simulink model "simulering_ROV_DP_model"  (R2020a)
settings: Solver=VariableStepAuto  StartTime=0.0  StopTime=t_sim  RelTol=1e-3
values from neighbouring files (symbols this model uses):
  B = [b11 b12 b13 b14 b15 b16 ... (first row only)    [constants.m]    (also in constants_dp_model.m; constants_model_coriolis.m; constants_process_model.m)
  B_psinv = B'/(B*B')    [constants_dp_model.m]    (also in constants_model_coriolis.m)
  d_11 = 250    [constants.m]    (also in constants_dp_model.m; constants_model_coriolis.m; constants_process_model.m)
  d_22 = 200    [constants.m]    (also in constants_dp_model.m; constants_model_coriolis.m; constants_process_model.m)
  d_33 = 175    [constants.m]    (also in constants_dp_model.m; constants_model_coriolis.m; constants_process_model.m)
  d_44 = 20    [constants.m]    (also in constants_dp_model.m = 15; constants_model_coriolis.m = 15; constants_process_model.m)
  g_z = 9.81    [run_simulation_FL_controller.m]    (also in run_simulation_PID_controller.m = 0.91; run_simulation_SM_controller.m = 0.91; run_simulation_STA_controller.m = 0.91; run_simulation_dp_model.m)
  gamma1 = 0.5    [run_simulation_dp_model.m]    (also in tuning_dp_model.m = 50)
  gamma2 = 0.5    [run_simulation_dp_model.m]    (also in tuning_dp_model.m = 35)
  k_d_psi = 2*m_44*zeta_d_psi*wn_psi-d_44    [run_simulation_PID_controller.m]    (also in run_simulation_SM_controller.m = 10; run_simulation_dp_model.m; run_simulation_feedback_linearizing.m = (2*1*k_p_psi*1-d33/(m_A33+m_RB33)); tuning_PID_controller.m = 2*m_66*zeta_d_psi*wn_psi-d_66)
  k_d_w = 2*m_33*zeta_d_heave*wn_heave-d_33    [run_simulation_FL_controller.m]    (also in run_simulation_dp_model.m; run_simulation_feedback_linearizing_second_try.m)
  k_i_psi = wn_psi/10*k_p_psi    [run_simulation_PID_controller.m]    (also in run_simulation_dp_model.m = 1/10*k_p_psi; tuning_PID_controller.m; tuning_dp_model.m = 0)
  k_i_w = wn_heave/10*k_p_w    [run_simulation_FL_controller.m]    (also in run_simulation_dp_model.m; run_simulation_feedback_linearizing_second_try.m)
  k_p_psi = wn_psi^2-lambda*k_p_r    [run_simulation_FL_controller.m]    (also in run_simulation_PID_controller.m = wn_psi^2*m_44; run_simulation_dp_model.m = wn_psi^2*m_44; run_simulation_feedback_linearizing.m = tau_r_max/deg2rad(45); run_simulation_feedback_linearizing_second_try.m = wn_psi^2*m_44)
  k_p_u = m_11*pole_u-d_11    [run_simulation_FL_controller.m]    (also in run_simulation_PID_controller.m = 10; run_simulation_dp_model.m = pole_u-d_11/m_11; run_simulation_feedback_linearizing.m = tau_u_max/100; run_simulation_feedback_linearizing_second_try.m = 1)
  k_p_v = m_22*pole_v-d_22    [run_simulation_FL_controller.m]    (also in run_simulation_PID_controller.m = 10; run_simulation_dp_model.m = pole_v-d_22/m_22; run_simulation_feedback_linearizing.m = tau_v_max/100; run_simulation_feedback_linearizing_second_try.m = 1)
  k_p_w = wn_heave^2*m_33    [run_simulation_FL_controller.m]    (also in run_simulation_dp_model.m; run_simulation_feedback_linearizing_second_try.m)
  m_11 = m_RB11+m_A11    (= 144)    [constants.m]    (also in constants_dp_model.m; constants_model_coriolis.m; constants_process_model.m)
  m_22 = m_RB22+m_A22    (= 162)    [constants.m]    (also in constants_dp_model.m; constants_model_coriolis.m; constants_process_model.m)
  m_A11 = 54    [constants.m]    (also in constants_dp_model.m; constants_model_coriolis.m; constants_process_model.m)
  m_A22 = 72    [constants.m]    (also in constants_dp_model.m; constants_model_coriolis.m; constants_process_model.m)
  m_A33 = 360    [constants.m]    (also in constants_dp_model.m; constants_model_coriolis.m; constants_process_model.m)
  m_A44 = 11    [constants.m]    (also in constants_dp_model.m = 5.2; constants_model_coriolis.m = 5.2; constants_process_model.m)
  m_RB11 = 90    [constants.m]    (also in constants_dp_model.m; constants_model_coriolis.m; constants_process_model.m)
  m_RB22 = 90    [constants.m]    (also in constants_dp_model.m; constants_model_coriolis.m; constants_process_model.m)
  m_RB33 = 90    [constants.m]    (also in constants_dp_model.m; constants_model_coriolis.m; constants_process_model.m)
  m_RB44 = 10    [constants.m]    (also in constants_dp_model.m = 13; constants_model_coriolis.m = 13; constants_process_model.m)
  omega_ref = 1.5    [run_simulation.m]    (also in run_simulation_FL_controller.m = 0.4; run_simulation_PID_controller.m = 0.4; run_simulation_SM_controller.m; run_simulation_STA_controller.m)
  psi0 = deg2rad(psi0)    [constants.m]    (also in constants_dp_model.m; constants_model_coriolis.m; constants_process_model.m)
  psi_r1 = deg2rad(psi_r1)    [run_simulation.m]    (also in run_simulation_FL_controller.m = 45; run_simulation_PID_controller.m = 45; run_simulation_SM_controller.m; run_simulation_STA_controller.m)
  psi_r2 = deg2rad(psi_r2)    [run_simulation.m]    (also in run_simulation_FL_controller.m = 90; run_simulation_PID_controller.m = 90; run_simulation_SM_controller.m; run_simulation_STA_controller.m)
  r0 = 0    [constants.m]    (also in constants_dp_model.m; constants_model_coriolis.m; constants_process_model.m)
  T_ref = 0.2    [run_simulation.m]    (also in run_simulation_FL_controller.m; run_simulation_PID_controller.m; run_simulation_SM_controller.m; run_simulation_STA_controller.m)
  tau_r_max = sqrt(torque_co'*torque_co)    [constants.m]    (also in constants_dp_model.m; constants_model_coriolis.m; constants_process_model.m; run_simulation_feedback_linearizing.m = sqrt(torque_co'*torque_co)/(m_A33+m_RB33))
  tau_u_max = (F_max*cos(alpha1)+F_max*cos(alpha2)+F_max*cos(alpha3)+F_max*cos(alpha4))    [constants.m]    (also in constants_dp_model.m; constants_model_coriolis.m; constants_process_model.m; run_simulation_feedback_linearizing.m = (F_max*cos(alpha1)+F_max*cos(alpha2)+F_max*cos(alpha3)+F_max)
  tau_v_max = (F_max*sin(alpha1)-F_max*sin(alpha2)+F_max*sin(alpha3)-F_max*sin(alpha4))    [constants.m]    (also in constants_dp_model.m; constants_model_coriolis.m; constants_process_model.m; run_simulation_feedback_linearizing.m = (F_max*sin(alpha1)-F_max*sin(alpha2)+F_max*sin(alpha3)-F_max)
  tau_w_max = 2*F_max    (= 240)    [constants.m]    (also in constants_dp_model.m; constants_model_coriolis.m; constants_process_model.m)
  u0 = 0    [constants.m]    (also in constants_dp_model.m; constants_model_coriolis.m; constants_process_model.m)
  u_r = 0.14    [run_simulation.m]    (also in run_simulation_FL_controller.m = 0.2; run_simulation_PID_controller.m = 0.2; run_simulation_SM_controller.m; run_simulation_STA_controller.m)
  v0 = 0    [constants.m]    (also in constants_dp_model.m; constants_model_coriolis.m; constants_process_model.m)
  v_r = 0.14    [run_simulation.m]    (also in run_simulation_FL_controller.m = 0; run_simulation_PID_controller.m = 0; run_simulation_SM_controller.m; run_simulation_STA_controller.m)
  V_x = 1    [constants.m]    (also in constants_process_model.m; run_simulation_FL_controller.m = 0.25; run_simulation_PID_controller.m = 0.25; run_simulation_dp_model.m = 0.25)
  V_y = 0    [constants.m]    (also in constants_process_model.m; run_simulation_FL_controller.m = -0.6; run_simulation_PID_controller.m = -0.6; run_simulation_dp_model.m = -0.6)
  w0 = 0    [constants.m]    (also in constants_dp_model.m; constants_model_coriolis.m; constants_process_model.m)
  x0 = -2*50    (= -100)    [constants.m]    (also in constants_dp_model.m = 0; constants_model_coriolis.m = 0; constants_process_model.m = 0)
  y0 = 0    [constants.m]    (also in constants_dp_model.m; constants_model_coriolis.m; constants_process_model.m)
  z0 = 0    [constants.m]    (also in constants_dp_model.m; constants_model_coriolis.m; constants_process_model.m)
  z_r = 10    [run_simulation.m]    (also in run_simulation_FL_controller.m = 1; run_simulation_PID_controller.m = 1; run_simulation_SM_controller.m; run_simulation_STA_controller.m)
  zeta_ref = 1    [run_simulation.m]    (also in run_simulation_FL_controller.m; run_simulation_PID_controller.m; run_simulation_SM_controller.m; run_simulation_STA_controller.m)
settings Model: Creator=kenng  LastModifiedBy=kenng

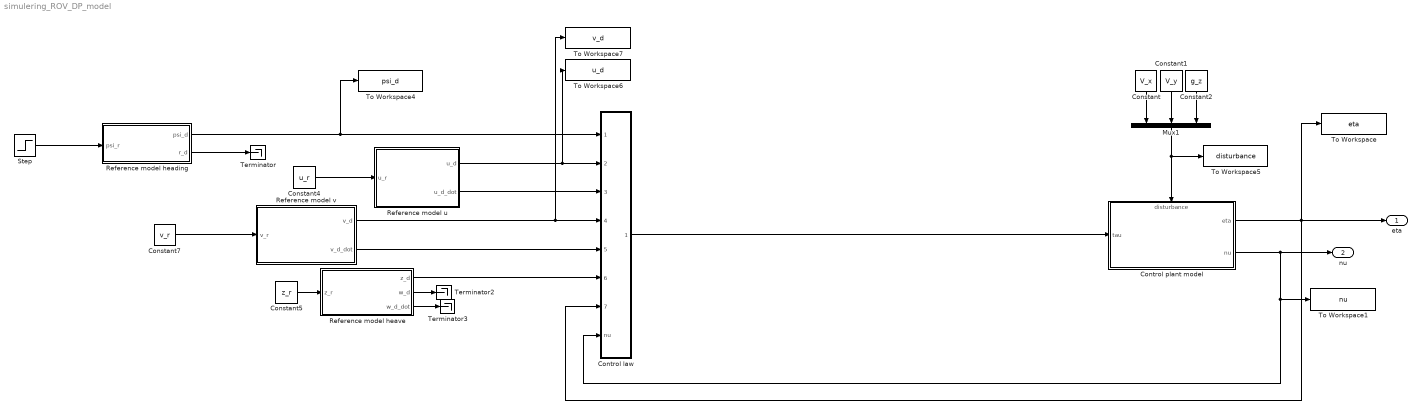
== system simulering_ROV_DP_model ==
  Constant : Constant  Value=V_x
  Constant1 : Constant  Value=V_y
  Constant2 : Constant  Value=g_z
  Constant4 : Constant  Value=u_r
  Constant5 : Constant  Value=z_r
  Constant7 : Constant  Value=v_r
  Control law : Subsystem
  Control plant model : Subsystem
      settings: PortSchema="{\"entries\":[{\"content\":{\"sides\":[{\"content\":{\"connectorIds\":[\"In1\"]},\"type\":\"ConnectorPlacement.EquallySpacedRectSide\",\"uuid\":\"e717a587-3200-458e-ba24-dd41565550b9\"},{\"content\":{\"connectorIds\":[\"Out1\",\"Out2\"],\"side\":\"RIGHT\"},\"type\":\"ConnectorPlacement.EquallySpacedRectSide\",\"uuid\":\"302c9cc9-c34e-45c2-bf93-40982187bd66\"},{\"content\":{\"connectorIds\":[\"In2\"],\"side\":\"TOP\"},\"type\":\"ConnectorPlacement.EquallySpacedRectSide\",\"uuid\":\"4b1c13ad-6fa1-447d-8a08-ad292496a8ea\"}]},\"type\":\"ConnectorPlacement.EquallySpacedConnector\",\"uuid\":\"78ff5622-69b9-4402-ac71-5e2cc2861626\"}],\"packageUris\":[\"http://schema.mathworks.com/mf0/Connector/19700101\"],\"version\":\"1.0\"}"
  Mux1 : Mux  Inputs=3
  Reference model heading : Subsystem
  Reference model heave : Subsystem
  Reference model u : Subsystem
  Reference model v : Subsystem
  Step : Step  Time=1000  Before=deg2rad(psi_r1)  After=deg2rad(psi_r2)  SampleTime=0
  Terminator : Terminator
  Terminator2 : Terminator
  Terminator3 : Terminator
  To Workspace : ToWorkspace  VariableName=eta  SaveFormat=Structure With Time  SampleTime=-1
  To Workspace1 : ToWorkspace  VariableName=nu  SaveFormat=Structure With Time  SampleTime=-1
  To Workspace4 : ToWorkspace  VariableName=psi_d  SaveFormat=Structure With Time  SampleTime=-1
  To Workspace5 : ToWorkspace  VariableName=disturbance  SaveFormat=Structure With Time  SampleTime=-1
  To Workspace6 : ToWorkspace  VariableName=u_d  SaveFormat=Structure With Time  SampleTime=-1
  To Workspace7 : ToWorkspace  VariableName=v_d  SaveFormat=Structure With Time  SampleTime=-1
  eta : Outport
  nu : Outport  Port=2
  wires:
  Control plant model/1(eta) -> Control law/7(eta), eta/1, To Workspace/1
  Control plant model/2(nu) -> nu/1, To Workspace1/1, Control law/8(nu)
  Mux1/1 -> Control plant model/2(disturbance), To Workspace5/1
  Reference model heading/1(psi_d) -> Control law/1(psi_d), To Workspace4/1
  Constant/1 -> Mux1/1
  Constant1/1 -> Mux1/2
  Constant2/1 -> Mux1/3
  Reference model heave/1(z_d) -> Control law/6(z_d)
  Control law/1(tau) -> Control plant model/1(tau)
  Step/1 -> Reference model heading/1(psi_r)
  Reference model heading/2(r_d) -> Terminator/1
  Constant4/1 -> Reference model u/1(u_r)
  Reference model heave/3(w_d_dot) -> Terminator3/1
  Reference model heave/2(w_d) -> Terminator2/1
  Constant5/1 -> Reference model heave/1(z_r)
  Constant7/1 -> Reference model v/1(v_r)
  Reference model u/1(u_d) -> To Workspace6/1, Control law/2(u_d)
  Reference model u/2(u_d_dot) -> Control law/3(u_d_dot)
  Reference model v/1(v_d) -> To Workspace7/1, Control law/4(v_d)
  Reference model v/2(v_d_dot) -> Control law/5(v_d_dot)

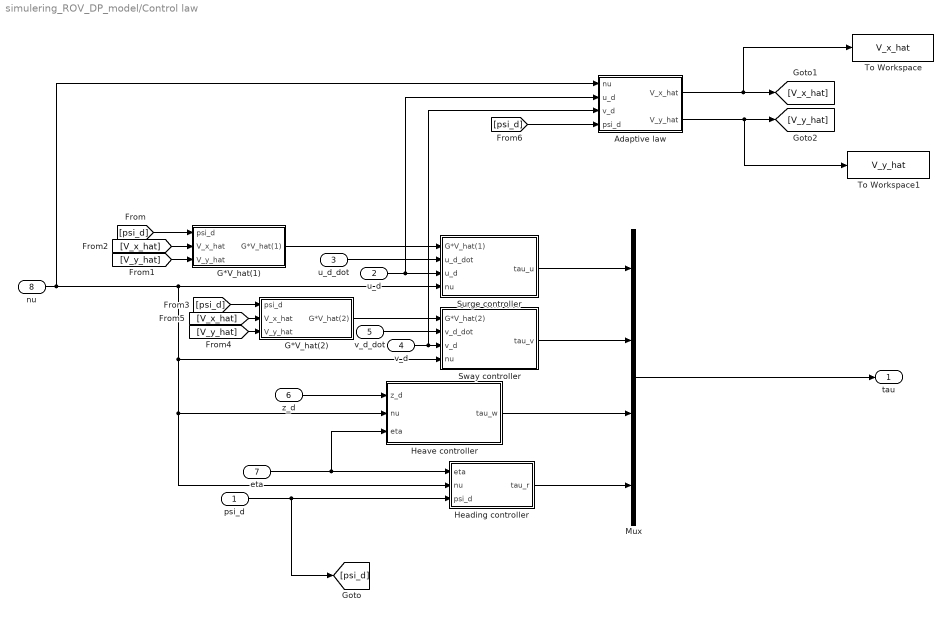
== system simulering_ROV_DP_model/Control law ==
  psi_d : Inport
  u_d : Inport  Port=2
  u_d_dot : Inport  Port=3
  v_d : Inport  Port=4
  v_d_dot : Inport  Port=5
  z_d : Inport  Port=6
  eta : Inport  Port=7
  nu : Inport  Port=8
  Adaptive law : Subsystem
  G*V_hat(1) : Subsystem
  G*V_hat(2) : Subsystem
  Heading controller : Subsystem
  Heave controller : Subsystem
  Mux : Mux
  Surge controller : Subsystem
  Sway controller : Subsystem
  To Workspace : ToWorkspace  VariableName=V_x_hat  SaveFormat=Structure With Time  SampleTime=-1
  To Workspace1 : ToWorkspace  VariableName=V_y_hat  SaveFormat=Structure With Time  SampleTime=-1
  tau : Outport
  wires:
  Surge controller/1(tau_u) -> Mux/1
  Sway controller/1(tau_v) -> Mux/2
  Heave controller/1(tau_w) -> Mux/3
  Mux/1 -> tau/1
  Heading controller/1(tau_r) -> Mux/4
  nu/1 -> Adaptive law/1(nu), Sway controller/4(nu), Heading controller/2(nu), Heave controller/2(nu), Surge controller/4(nu)
  eta/1 -> Heading controller/1(eta), Heave controller/3(eta)
  psi_d/1 -> [psi_d], Heading controller/3(psi_d)
  [V_y_hat] -> G*V_hat(1)/3(V_y_hat)
  [V_x_hat] -> G*V_hat(1)/2(V_x_hat)
  [psi_d] -> G*V_hat(1)/1(psi_d)
  G*V_hat(1)/1(G*V_hat(1)) -> Surge controller/1(G*V_hat(1))
  [psi_d] -> G*V_hat(2)/1(psi_d)
  [V_y_hat] -> G*V_hat(2)/3(V_y_hat)
  [V_x_hat] -> G*V_hat(2)/2(V_x_hat)
  G*V_hat(2)/1(G*V_hat(2)) -> Sway controller/1(G*V_hat(2))
  u_d/1 -> Adaptive law/2(u_d), Surge controller/3(u_d)
  u_d_dot/1 -> Surge controller/2(u_d_dot)
  v_d_dot/1 -> Sway controller/2(v_d_dot)
  v_d/1 -> Adaptive law/3(v_d), Sway controller/3(v_d)
  Adaptive law/1(V_x_hat) -> To Workspace/1, [V_x_hat]
  Adaptive law/2(V_y_hat) -> To Workspace1/1, [V_y_hat]
  [psi_d] -> Adaptive law/4(psi_d)
  z_d/1 -> Heave controller/1(z_d)

== system simulering_ROV_DP_model/Control plant model ==
  note: tau: 4x1 vector = [surge sway heave yaw]^T
  note: Disturbance: 3x1 vector = [Vx Vy gz]^t
  tau : Inport
  disturbance : Inport  Port=2
  Demux : Demux
  Kinematics : Subsystem
  Kinetics : Subsystem
  Terminator : Terminator
  Terminator1 : Terminator
  Terminator2 : Terminator
  Thruster saturation : Subsystem
  To Workspace2 : ToWorkspace  VariableName=tau_unsat  SaveFormat=Structure With Time  SampleTime=-1
  To Workspace3 : ToWorkspace  VariableName=tau_sat  SaveFormat=Structure With Time  SampleTime=-1
  eta : Outport
  nu : Outport  Port=2
  wires:
  Kinetics/1(nu) -> nu/1, Kinematics/1(nu)
  Demux/4 -> Kinetics/3(psi)
  Demux/2 -> Terminator1/1
  Kinematics/1(eta) -> eta/1, Demux/1
  Demux/1 -> Terminator/1
  Demux/3 -> Terminator2/1
  disturbance/1 -> Kinetics/1(disturbance)
  tau/1 -> To Workspace2/1, Thruster saturation/1(tau_unsat)
  Thruster saturation/1(tau_sat) -> To Workspace3/1, Kinetics/2(tau)

== system simulering_ROV_DP_model/Reference model heading ==
  note: psi_r
  note: psi_d
  note: r_d
  note: a_d
  psi_r : Inport
  Gain : Gain  Gain=(2*zeta_ref+1)*omega_ref
  Gain1 : Gain  Gain=(2*zeta_ref+1)*omega_ref^2
  Gain2 : Gain  Gain=omega_ref^3
  Integrator : Integrator
  Integrator1 : Integrator
  Integrator2 : Integrator
  Saturation : Saturate  UpperLimit=tau_r_max/(m_RB11*0.2^2)  LowerLimit=-tau_r_max/(m_RB11*0.2^2)
  Sum : Sum  Inputs=|+-
  Sum1 : Sum  Inputs=-+|
  Sum2 : Sum  Inputs=-+|
  psi_d : Outport
  r_d : Outport  Port=2
  wires:
  Sum1/1 -> Integrator1/1
  Sum2/1 -> Gain2/1
  Integrator2/1 -> psi_d/1, Sum2/1
  Sum/1 -> Sum1/2
  Saturation/1 -> Gain/1, Integrator/1
  Integrator/1 -> r_d/1, Gain1/1, Integrator2/1
  Gain2/1 -> Sum/1
  Gain/1 -> Sum/2
  Gain1/1 -> Sum1/1
  Integrator1/1 -> Saturation/1
  psi_r/1 -> Sum2/2

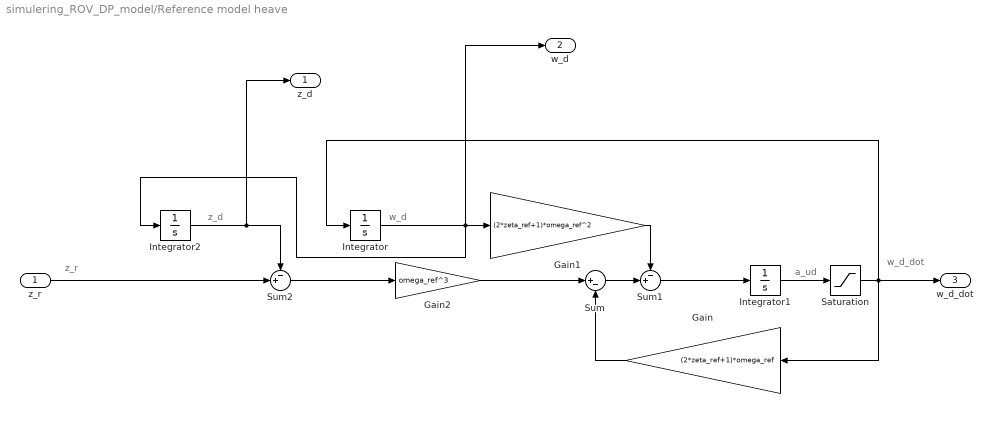
== system simulering_ROV_DP_model/Reference model heave ==
  note: w_d_dot
  note: z_r
  note: z_d
  note: w_d
  note: a_ud
  z_r : Inport
  Gain : Gain  Gain=(2*zeta_ref+1)*omega_ref
  Gain1 : Gain  Gain=(2*zeta_ref+1)*omega_ref^2
  Gain2 : Gain  Gain=omega_ref^3
  Integrator : Integrator
  Integrator1 : Integrator
  Integrator2 : Integrator
  Saturation : Saturate  UpperLimit=tau_w_max/m_RB11  LowerLimit=-tau_w_max/m_RB11
  Sum : Sum  Inputs=|+-
  Sum1 : Sum  Inputs=-+|
  Sum2 : Sum  Inputs=-+|
  z_d : Outport
  w_d : Outport  Port=2
  w_d_dot : Outport  Port=3
  wires:
  Sum1/1 -> Integrator1/1
  Sum2/1 -> Gain2/1
  Integrator2/1 -> z_d/1, Sum2/1
  Sum/1 -> Sum1/2
  Saturation/1 -> Integrator/1, w_d_dot/1, Gain/1
  Gain2/1 -> Sum/1
  Gain/1 -> Sum/2
  Gain1/1 -> Sum1/1
  Integrator1/1 -> Saturation/1
  z_r/1 -> Sum2/2
  Integrator/1 -> w_d/1, Gain1/1, Integrator2/1

== system simulering_ROV_DP_model/Reference model u ==
  note: u_r
  u_r : Inport
  Gain : Gain  Gain=1/T_ref
  Integrator : Integrator
  Saturation : Saturate  UpperLimit=tau_u_max/m_RB11  LowerLimit=-tau_u_max/m_RB11
  Sum : Sum  Inputs=|+-
  u_d : Outport
  u_d_dot : Outport  Port=2
  wires:
  u_r/1 -> Sum/1
  Sum/1 -> Gain/1
  Integrator/1 -> u_d/1, Sum/2
  Gain/1 -> Saturation/1
  Saturation/1 -> u_d_dot/1, Integrator/1

== system simulering_ROV_DP_model/Reference model v ==
  note: v_r
  v_r : Inport
  Gain : Gain  Gain=1/T_ref
  Integrator : Integrator
  Saturation : Saturate
  Saturation1 : Saturate  UpperLimit=tau_v_max/m_RB11  LowerLimit=-tau_v_max/m_RB11
  Sum : Sum  Inputs=|+-
  v_d : Outport
  v_d_dot : Outport  Port=2
  wires:
  v_r/1 -> Sum/1
  Sum/1 -> Gain/1
  Integrator/1 -> Saturation/1
  Gain/1 -> Saturation1/1
  Saturation/1 -> v_d/1, Sum/2
  Saturation1/1 -> v_d_dot/1, Integrator/1

== system simulering_ROV_DP_model/Control law/Adaptive law ==
  nu : Inport
  u_d : Inport  Port=2
  v_d : Inport  Port=3
  psi_d : Inport  Port=4
  Subsystem : Subsystem
  v_x_hat : Subsystem
  v_y_hat : Subsystem
  V_x_hat : Outport
  V_y_hat : Outport  Port=2
  wires:
  nu/1 -> Subsystem/1(nu)
  Subsystem/2(v_tilde) -> v_y_hat/3(v_tilde), v_x_hat/3(v_tilde)
  psi_d/1 -> v_y_hat/1(psi_d), v_x_hat/1(psi_d)
  Subsystem/1(u_tilde) -> v_x_hat/2(u_tilde), v_y_hat/2(u_tilde)
  v_d/1 -> Subsystem/3(v_d)
  v_x_hat/1(V_x_hat) -> V_x_hat/1
  u_d/1 -> Subsystem/2(u_d)
  v_y_hat/1(V_y_hat) -> V_y_hat/1

== system simulering_ROV_DP_model/Control law/G*V_hat(1) ==
  psi_d : Inport
  V_x_hat : Inport  Port=2
  V_y_hat : Inport  Port=3
  Cos : Trigonometry  Operator=cos
  Gain : Gain  Gain=d_11/m_11
  Gain1 : Gain  Gain=d_11/m_11
  Product : Product
  Product1 : Product
  Sin : Trigonometry
  Sum : Sum  Inputs=|++
  G*V_hat(1) : Outport
  wires:
  Gain1/1 -> Product1/1
  Sin/1 -> Gain1/1
  psi_d/1 -> Sin/1, Cos/1
  Product/1 -> Sum/1
  Product1/1 -> Sum/2
  V_x_hat/1 -> Product/1
  Cos/1 -> Gain/1
  V_y_hat/1 -> Product1/2
  Gain/1 -> Product/2
  Sum/1 -> G*V_hat(1)/1

== system simulering_ROV_DP_model/Control law/G*V_hat(2) ==
  psi_d : Inport
  V_x_hat : Inport  Port=2
  V_y_hat : Inport  Port=3
  Cos : Trigonometry  Operator=cos
  Gain : Gain  Gain=d_22/m_22
  Gain1 : Gain  Gain=d_22/m_22
  Product : Product
  Product1 : Product
  Sin : Trigonometry
  Sum : Sum  Inputs=|+-
  G*V_hat(2) : Outport
  wires:
  Sum/1 -> G*V_hat(2)/1
  Gain/1 -> Product/2
  V_x_hat/1 -> Product1/2
  Cos/1 -> Gain/1
  V_y_hat/1 -> Product/1
  Product1/1 -> Sum/2
  Product/1 -> Sum/1
  psi_d/1 -> Cos/1, Sin/1
  Sin/1 -> Gain1/1
  Gain1/1 -> Product1/1

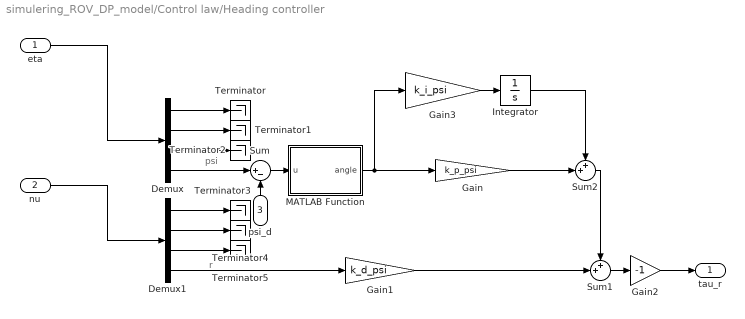
== system simulering_ROV_DP_model/Control law/Heading controller ==
  note: r
  note: psi
  eta : Inport
  nu : Inport  Port=2
  psi_d : Inport  Port=3
  Demux : Demux
  Demux1 : Demux
  Gain : Gain  Gain=k_p_psi
  Gain1 : Gain  Gain=k_d_psi
  Gain2 : Gain  Gain=-1
  Gain3 : Gain  Gain=k_i_psi
  Integrator : Integrator
  MATLAB Function : MATLAB Function  TreatAsAtomicUnit=on
  Sum : Sum  Inputs=|+-
  Sum1 : Sum  Inputs=++|
  Sum2 : Sum  Inputs=++|
  Terminator{,1..5} (6 alike) : Terminator
  tau_r : Outport
  wires:
  Demux1/2 -> Terminator4/1
  Demux/3 -> Terminator2/1
  Demux1/1 -> Terminator3/1
  Gain1/1 -> Sum1/2
  Demux/1 -> Terminator/1
  Sum1/1 -> Gain2/1
  Demux/2 -> Terminator1/1
  Demux1/4 -> Gain1/1
  Demux1/3 -> Terminator5/1
  Demux/4 -> Sum/1
  Sum/1 -> MATLAB Function/1(u)
  eta/1 -> Demux/1
  Gain2/1 -> tau_r/1
  nu/1 -> Demux1/1
  psi_d/1 -> Sum/2
  MATLAB Function/1(angle) -> Gain/1, Gain3/1
  Gain3/1 -> Integrator/1
  Gain/1 -> Sum2/2
  Sum2/1 -> Sum1/1
  Integrator/1 -> Sum2/1

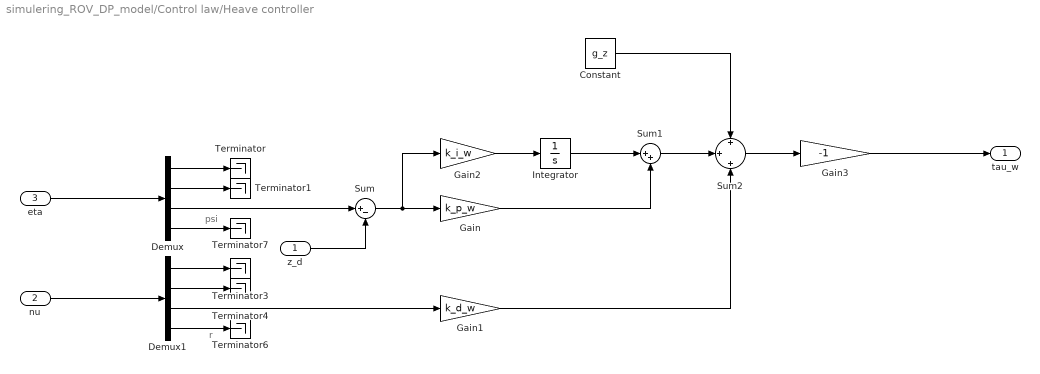
== system simulering_ROV_DP_model/Control law/Heave controller ==
  note: r
  note: psi
  z_d : Inport
  nu : Inport  Port=2
  eta : Inport  Port=3
  Constant : Constant  Value=g_z
  Demux : Demux
  Demux1 : Demux
  Gain : Gain  Gain=k_p_w
  Gain1 : Gain  Gain=k_d_w
  Gain2 : Gain  Gain=k_i_w
  Gain3 : Gain  Gain=-1
  Integrator : Integrator
  Sum : Sum  Inputs=|+-
  Sum1 : Sum  Inputs=|++
  Sum2 : Sum  Inputs=+|+|+
  Terminator{,1,3..4,6..7} (6 alike) : Terminator
  tau_w : Outport
  wires:
  Demux1/2 -> Terminator4/1
  Demux/1 -> Terminator/1
  eta/1 -> Demux/1
  Demux/2 -> Terminator1/1
  Demux1/1 -> Terminator3/1
  Demux/3 -> Sum/1
  nu/1 -> Demux1/1
  Demux1/4 -> Terminator6/1
  Demux/4 -> Terminator7/1
  z_d/1 -> Sum/2
  Sum/1 -> Gain2/1, Gain/1
  Demux1/3 -> Gain1/1
  Gain2/1 -> Integrator/1
  Integrator/1 -> Sum1/1
  Gain/1 -> Sum1/2
  Sum2/1 -> Gain3/1
  Gain3/1 -> tau_w/1
  Gain1/1 -> Sum2/3
  Sum1/1 -> Sum2/2
  Constant/1 -> Sum2/1

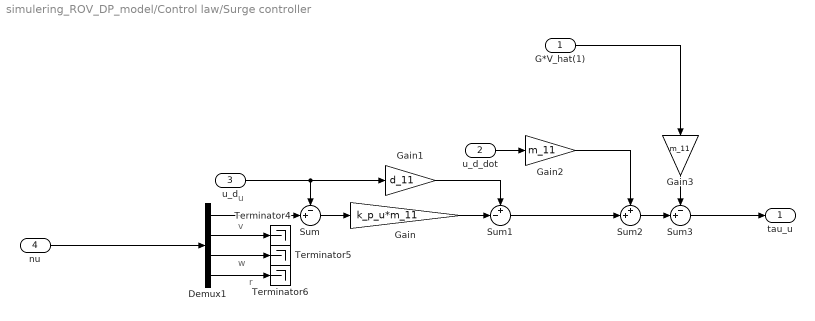
== system simulering_ROV_DP_model/Control law/Surge controller ==
  note: u
  note: r
  note: v
  note: w
  G*V_hat(1) : Inport
  u_d_dot : Inport  Port=2
  u_d : Inport  Port=3
  nu : Inport  Port=4
  Demux1 : Demux
  Gain : Gain  Gain=k_p_u*m_11
  Gain1 : Gain  Gain=d_11
  Gain2 : Gain  Gain=m_11
  Gain3 : Gain  Gain=m_11
  Sum : Sum  Inputs=-+|
  Sum1 : Sum  Inputs=+-|
  Sum2 : Sum  Inputs=++|
  Sum3 : Sum  Inputs=-+|
  Terminator4 : Terminator
  Terminator5 : Terminator
  Terminator6 : Terminator
  tau_u : Outport
  wires:
  Demux1/2 -> Terminator4/1
  Demux1/4 -> Terminator6/1
  Demux1/1 -> Sum/2
  nu/1 -> Demux1/1
  Demux1/3 -> Terminator5/1
  u_d/1 -> Gain1/1, Sum/1
  Sum/1 -> Gain/1
  Gain/1 -> Sum1/2
  Gain1/1 -> Sum1/1
  Sum1/1 -> Sum2/2
  u_d_dot/1 -> Gain2/1
  Gain2/1 -> Sum2/1
  Sum2/1 -> Sum3/2
  Gain3/1 -> Sum3/1
  G*V_hat(1)/1 -> Gain3/1
  Sum3/1 -> tau_u/1

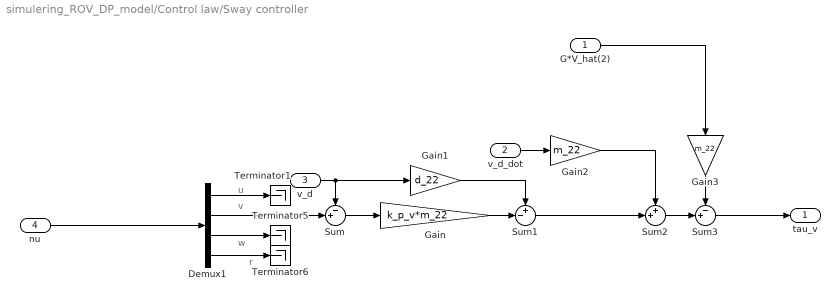
== system simulering_ROV_DP_model/Control law/Sway controller ==
  note: w
  note: v
  note: r
  note: u
  G*V_hat(2) : Inport
  v_d_dot : Inport  Port=2
  v_d : Inport  Port=3
  nu : Inport  Port=4
  Demux1 : Demux
  Gain : Gain  Gain=k_p_v*m_22
  Gain1 : Gain  Gain=d_22
  Gain2 : Gain  Gain=m_22
  Gain3 : Gain  Gain=m_22
  Sum : Sum  Inputs=-+|
  Sum1 : Sum  Inputs=+-|
  Sum2 : Sum  Inputs=++|
  Sum3 : Sum  Inputs=-+|
  Terminator1 : Terminator
  Terminator5 : Terminator
  Terminator6 : Terminator
  tau_v : Outport
  wires:
  Sum3/1 -> tau_v/1
  G*V_hat(2)/1 -> Gain3/1
  Gain3/1 -> Sum3/1
  Sum2/1 -> Sum3/2
  Gain2/1 -> Sum2/1
  v_d_dot/1 -> Gain2/1
  Sum1/1 -> Sum2/2
  Gain1/1 -> Sum1/1
  Gain/1 -> Sum1/2
  Sum/1 -> Gain/1
  v_d/1 -> Sum/1, Gain1/1
  Demux1/3 -> Terminator5/1
  nu/1 -> Demux1/1
  Demux1/4 -> Terminator6/1
  Demux1/2 -> Sum/2
  Demux1/1 -> Terminator1/1

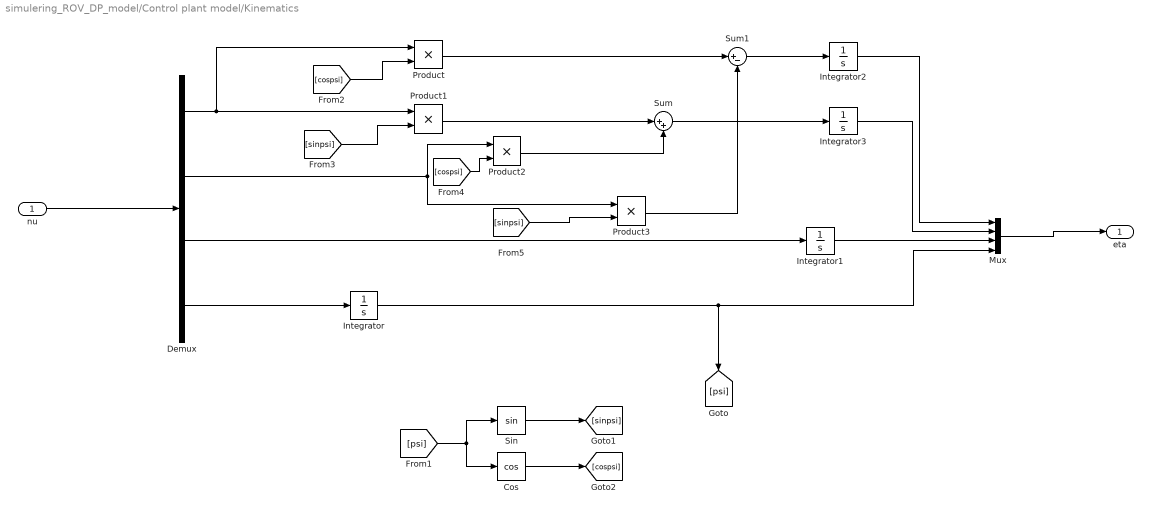
== system simulering_ROV_DP_model/Control plant model/Kinematics ==
  nu : Inport
  Cos : Trigonometry  Operator=cos
  Demux : Demux
  Integrator : Integrator  InitialCondition=psi0
  Integrator1 : Integrator  InitialCondition=z0
  Integrator2 : Integrator  InitialCondition=x0
  Integrator3 : Integrator  InitialCondition=y0
  Mux : Mux
  Product{,1..3} (4 alike) : Product
  Sin : Trigonometry
  Sum : Sum  Inputs=|++
  Sum1 : Sum  Inputs=|+-
  eta : Outport
  wires:
  Sin/1 -> [sinpsi]
  Demux/3 -> Integrator1/1
  Demux/1 -> Product1/1, Product/1
  Demux/2 -> Product3/1, Product2/1
  [sinpsi] -> Product3/2
  [psi] -> Sin/1, Cos/1
  [cospsi] -> Product2/2
  Cos/1 -> [cospsi]
  Product1/1 -> Sum/1
  Integrator/1 -> Mux/4, [psi]
  [sinpsi] -> Product1/2
  Product/1 -> Sum1/1
  Sum1/1 -> Integrator2/1
  Demux/4 -> Integrator/1
  Sum/1 -> Integrator3/1
  [cospsi] -> Product/2
  nu/1 -> Demux/1
  Product2/1 -> Sum/2
  Product3/1 -> Sum1/2
  Integrator3/1 -> Mux/2
  Integrator1/1 -> Mux/3
  Integrator2/1 -> Mux/1
  Mux/1 -> eta/1

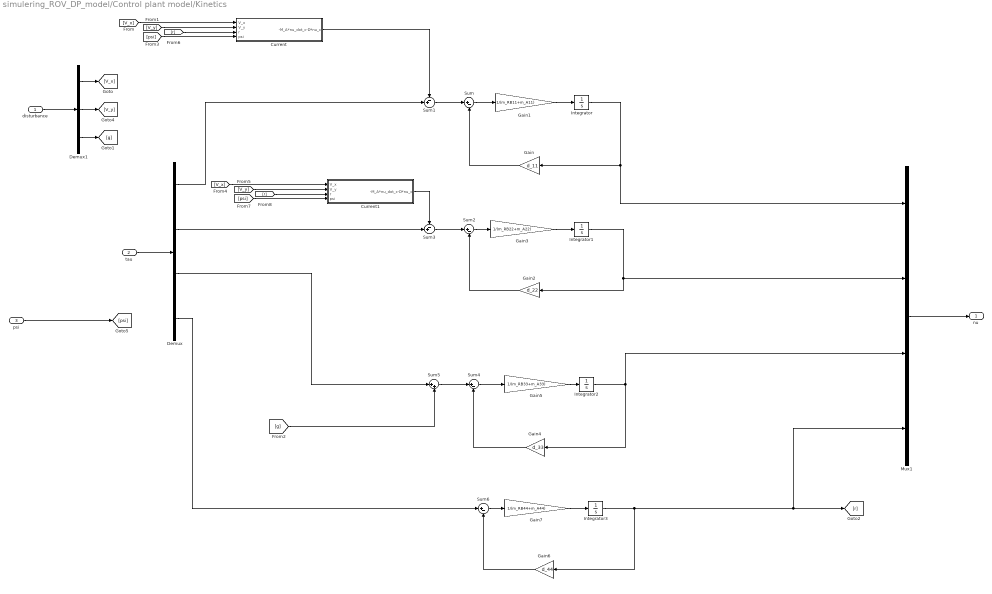
== system simulering_ROV_DP_model/Control plant model/Kinetics ==
  disturbance : Inport
  tau : Inport  Port=2
  psi : Inport  Port=3
  Current : Subsystem
  Current1 : Subsystem
  Demux : Demux
  Demux1 : Demux  Outputs=3
  Gain : Gain  Gain=d_11
  Gain1 : Gain  Gain=1/(m_RB11+m_A11)
  Gain2 : Gain  Gain=d_22
  Gain3 : Gain  Gain=1/(m_RB22+m_A22)
  Gain4 : Gain  Gain=d_33
  Gain5 : Gain  Gain=1/(m_RB33+m_A33)
  Gain6 : Gain  Gain=d_44
  Gain7 : Gain  Gain=1/(m_RB44+m_A44)
  Integrator : Integrator  InitialCondition=u0
  Integrator1 : Integrator  InitialCondition=v0
  Integrator2 : Integrator  InitialCondition=w0
  Integrator3 : Integrator  InitialCondition=r0
  Mux1 : Mux
  Sum{,2,4,6} (4 alike) : Sum  Inputs=|+-
  Sum1 : Sum  Inputs=-+|
  Sum3 : Sum  Inputs=-+|
  Sum5 : Sum  Inputs=|++
  nu : Outport
  wires:
  Demux1/1 -> [V_x]
  Gain1/1 -> Integrator/1
  Sum/1 -> Gain1/1
  tau/1 -> Demux/1
  Integrator1/1 -> Gain2/1, Mux1/2
  Gain3/1 -> Integrator1/1
  Mux1/1 -> nu/1
  Demux/1 -> Sum1/2
  Integrator/1 -> Mux1/1, Gain/1
  Integrator2/1 -> Gain4/1, Mux1/3
  Gain5/1 -> Integrator2/1
  Demux1/3 -> [g]
  Sum3/1 -> Sum2/1
  Sum4/1 -> Gain5/1
  Gain2/1 -> Sum2/2
  Sum2/1 -> Gain3/1
  Gain/1 -> Sum/2
  Gain4/1 -> Sum4/2
  Demux/4 -> Sum6/1
  Sum1/1 -> Sum/1
  Gain6/1 -> Sum6/2
  Demux1/2 -> [V_y]
  [r] -> Current/3(r)
  Demux/2 -> Sum3/2
  Integrator3/1 -> [r], Mux1/4, Gain6/1
  disturbance/1 -> Demux1/1
  Sum6/1 -> Gain7/1
  Gain7/1 -> Integrator3/1
  psi/1 -> [psi]
  Current/1(-M_A*nu_dot_c-D*nu_c) -> Sum1/1
  [V_y] -> Current/2(V_y)
  [V_x] -> Current/1(V_x)
  [psi] -> Current/4(psi)
  [r] -> Current1/3(r)
  [psi] -> Current1/4(psi)
  [V_x] -> Current1/1(V_x)
  [V_y] -> Current1/2(V_y)
  Current1/1(-M_A*nu_dot_c-D*nu_c) -> Sum3/1
  [g] -> Sum5/2
  Demux/3 -> Sum5/1
  Sum5/1 -> Sum4/1

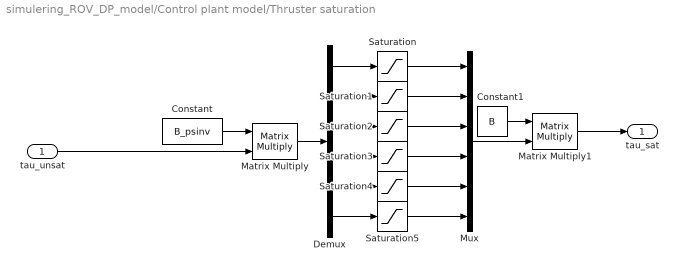
== system simulering_ROV_DP_model/Control plant model/Thruster saturation ==
  tau_unsat : Inport
  Constant : Constant  Value=B_psinv
  Constant1 : Constant  Value=B
  Demux : Demux  Outputs=6
  Matrix Multiply : Product  Multiplication=Matrix(*)
  Matrix Multiply1 : Product  Multiplication=Matrix(*)
  Mux : Mux  Inputs=6
  Saturation{,1..5} (6 alike) : Saturate  UpperLimit=120  LowerLimit=-120
  tau_sat : Outport
  wires:
  tau_unsat/1 -> Matrix Multiply/2
  Constant/1 -> Matrix Multiply/1
  Matrix Multiply/1 -> Demux/1
  Demux/2 -> Saturation1/1
  Demux/1 -> Saturation/1
  Demux/3 -> Saturation2/1
  Demux/4 -> Saturation3/1
  Demux/5 -> Saturation4/1
  Demux/6 -> Saturation5/1
  Saturation/1 -> Mux/1
  Saturation1/1 -> Mux/2
  Saturation2/1 -> Mux/3
  Saturation3/1 -> Mux/4
  Saturation4/1 -> Mux/5
  Saturation5/1 -> Mux/6
  Mux/1 -> Matrix Multiply1/2
  Constant1/1 -> Matrix Multiply1/1
  Matrix Multiply1/1 -> tau_sat/1

== system simulering_ROV_DP_model/Control law/Adaptive law/Subsystem ==
  note: u
  note: r
  note: w
  note: v
  nu : Inport
  u_d : Inport  Port=2
  v_d : Inport  Port=3
  Demux1 : Demux
  Sum : Sum  Inputs=|+-
  Sum1 : Sum  Inputs=|+-
  Terminator5 : Terminator
  Terminator6 : Terminator
  u_tilde : Outport
  v_tilde : Outport  Port=2
  wires:
  Sum1/1 -> u_tilde/1
  v_d/1 -> Sum/2
  Sum/1 -> v_tilde/1
  u_d/1 -> Sum1/2
  Demux1/2 -> Sum/1
  nu/1 -> Demux1/1
  Demux1/4 -> Terminator6/1
  Demux1/1 -> Sum1/1
  Demux1/3 -> Terminator5/1

== system simulering_ROV_DP_model/Control law/Adaptive law/v_x_hat ==
  psi_d : Inport
  u_tilde : Inport  Port=2
  v_tilde : Inport  Port=3
  Cos : Trigonometry  Operator=cos
  Gain : Gain  Gain=d_11/m_11
  Gain1 : Gain  Gain=d_22/m_22
  Gain2 : Gain  Gain=gamma1
  Integrator : Integrator
  Product : Product
  Product1 : Product
  Sin : Trigonometry
  Sum : Sum  Inputs=|+-
  V_x_hat : Outport
  wires:
  Sum/1 -> Gain2/1
  Gain/1 -> Product/2
  v_tilde/1 -> Product1/2
  Cos/1 -> Gain/1
  u_tilde/1 -> Product/1
  Product1/1 -> Sum/2
  Product/1 -> Sum/1
  psi_d/1 -> Cos/1, Sin/1
  Sin/1 -> Gain1/1
  Gain1/1 -> Product1/1
  Gain2/1 -> Integrator/1
  Integrator/1 -> V_x_hat/1

== system simulering_ROV_DP_model/Control law/Adaptive law/v_y_hat ==
  psi_d : Inport
  u_tilde : Inport  Port=2
  v_tilde : Inport  Port=3
  Cos : Trigonometry  Operator=cos
  Gain : Gain  Gain=d_22/m_22
  Gain1 : Gain  Gain=d_11/m_11
  Gain2 : Gain  Gain=gamma2
  Integrator : Integrator
  Product : Product
  Product1 : Product
  Sin : Trigonometry
  Sum : Sum  Inputs=|++
  V_y_hat : Outport
  wires:
  Gain1/1 -> Product1/1
  Sin/1 -> Gain1/1
  psi_d/1 -> Sin/1, Cos/1
  Product/1 -> Sum/1
  Product1/1 -> Sum/2
  v_tilde/1 -> Product/1
  Cos/1 -> Gain/1
  u_tilde/1 -> Product1/2
  Gain/1 -> Product/2
  Sum/1 -> Gain2/1
  Gain2/1 -> Integrator/1
  Integrator/1 -> V_y_hat/1

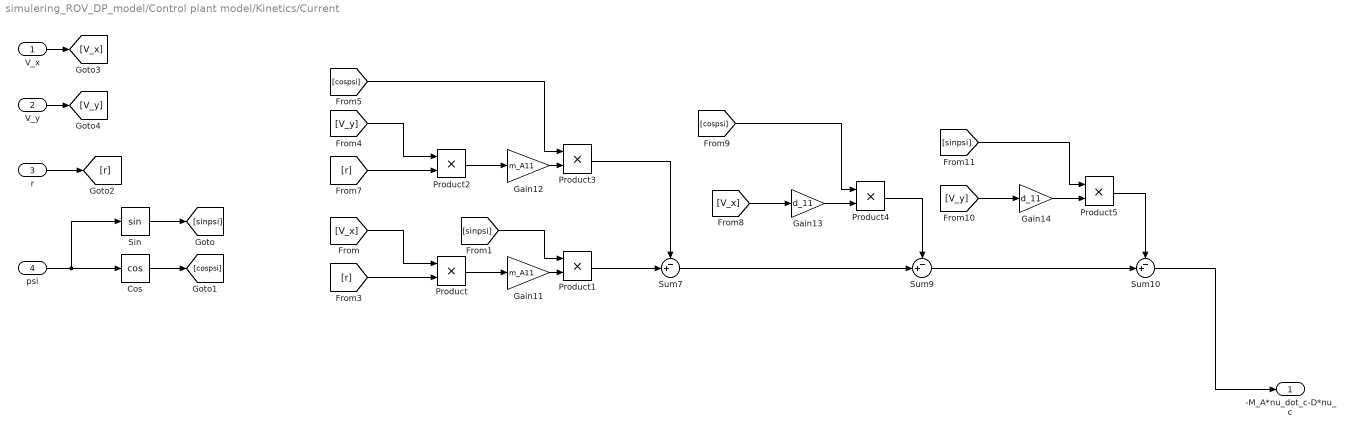
== system simulering_ROV_DP_model/Control plant model/Kinetics/Current ==
  V_x : Inport
  V_y : Inport  Port=2
  r : Inport  Port=3
  psi : Inport  Port=4
  Cos : Trigonometry  Operator=cos
  Gain11 : Gain  Gain=m_A11
  Gain12 : Gain  Gain=m_A11
  Gain13 : Gain  Gain=d_11
  Gain14 : Gain  Gain=d_11
  Product{,1..5} (6 alike) : Product
  Sin : Trigonometry
  Sum10 : Sum  Inputs=-+|
  Sum7 : Sum  Inputs=-+|
  Sum9 : Sum  Inputs=-+|
  -M_A*nu_dot_c-D*nu_c : Outport
  wires:
  Gain11/1 -> Product1/2
  Product2/1 -> Gain12/1
  [cospsi] -> Product3/1
  [r] -> Product2/2
  Gain13/1 -> Product4/2
  Product4/1 -> Sum9/1
  [V_x] -> Product/1
  Product3/1 -> Sum7/1
  Gain12/1 -> Product3/2
  Product/1 -> Gain11/1
  [V_y] -> Product2/1
  [r] -> Product/2
  Product1/1 -> Sum7/2
  [sinpsi] -> Product1/1
  Gain14/1 -> Product5/2
  [sinpsi] -> Product5/1
  Sum7/1 -> Sum9/2
  [cospsi] -> Product4/1
  [V_y] -> Gain14/1
  [V_x] -> Gain13/1
  Product5/1 -> Sum10/1
  Sum9/1 -> Sum10/2
  Sum10/1 -> -M_A*nu_dot_c-D*nu_c/1
  psi/1 -> Sin/1, Cos/1
  Sin/1 -> [sinpsi]
  Cos/1 -> [cospsi]
  r/1 -> [r]
  V_x/1 -> [V_x]
  V_y/1 -> [V_y]

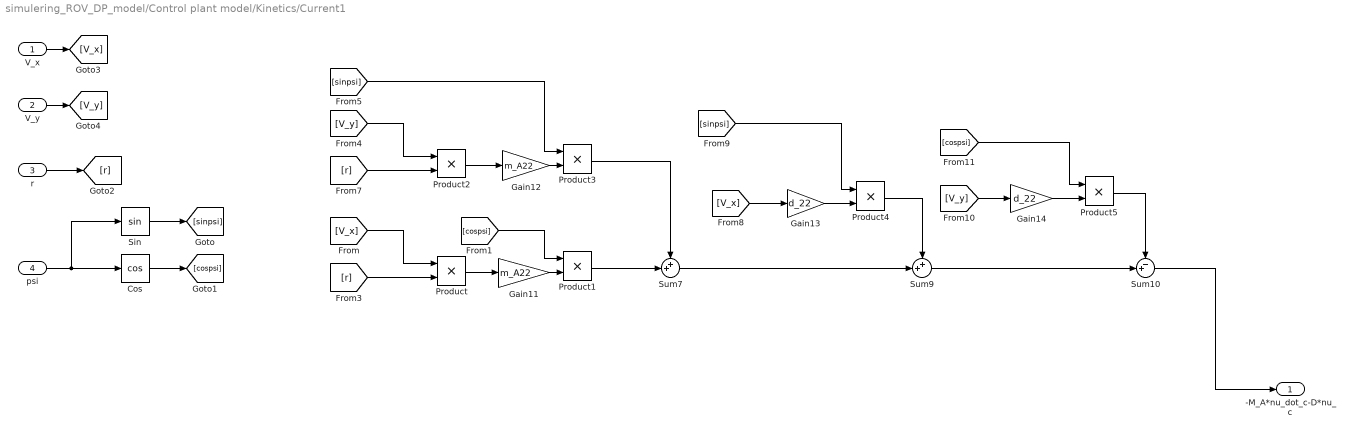
== system simulering_ROV_DP_model/Control plant model/Kinetics/Current1 ==
  V_x : Inport
  V_y : Inport  Port=2
  r : Inport  Port=3
  psi : Inport  Port=4
  Cos : Trigonometry  Operator=cos
  Gain11 : Gain  Gain=m_A22
  Gain12 : Gain  Gain=m_A22
  Gain13 : Gain  Gain=d_22
  Gain14 : Gain  Gain=d_22
  Product{,1..5} (6 alike) : Product
  Sin : Trigonometry
  Sum10 : Sum  Inputs=-+|
  Sum7 : Sum  Inputs=++|
  Sum9 : Sum  Inputs=++|
  -M_A*nu_dot_c-D*nu_c : Outport
  wires:
  Gain11/1 -> Product1/2
  Product2/1 -> Gain12/1
  [sinpsi] -> Product3/1
  [r] -> Product2/2
  Gain13/1 -> Product4/2
  Product4/1 -> Sum9/1
  [V_x] -> Product/1
  Product3/1 -> Sum7/1
  Gain12/1 -> Product3/2
  Product/1 -> Gain11/1
  [V_y] -> Product2/1
  [r] -> Product/2
  Product1/1 -> Sum7/2
  [cospsi] -> Product1/1
  Gain14/1 -> Product5/2
  [cospsi] -> Product5/1
  Sum7/1 -> Sum9/2
  [sinpsi] -> Product4/1
  [V_y] -> Gain14/1
  [V_x] -> Gain13/1
  Product5/1 -> Sum10/1
  Sum9/1 -> Sum10/2
  Sum10/1 -> -M_A*nu_dot_c-D*nu_c/1
  psi/1 -> Sin/1, Cos/1
  Sin/1 -> [sinpsi]
  Cos/1 -> [cospsi]
  r/1 -> [r]
  V_x/1 -> [V_x]
  V_y/1 -> [V_y]

== matlab function simulering_ROV_DP_model/Control law/Heading controller/MATLAB Function ==
  data: u input; angle output
function angle = fcn(u)
%#codegen

angle = ssa(u);
